simulink model "Phase 3 Onboard PFC Boost Charger-BMW i4 eDrive35 Gran Coupe Simulation"  (R2024b)
settings: Solver=VariableStepAuto  StartTime=0.0  StopTime=1  RelTol=1e-3
libraries: spsRMSLib x13, spsMeanLib x12, spsDiodeLib x9, spsCurrentMeasurementLib x5, spsMosfetLib x5, spsSeriesRLCBranchLib x5, spsVoltageMeasurementLib x5, slpidlib x2, spsPWMGeneratorDCDCLib x2, spsACVoltageSourceLib x1, spsLinearTransformerLib x1, sps_lib x1
settings Model: Creator=17249  LastModifiedBy=kunas
settings RTWCC: GPUComputeCapability=3.5

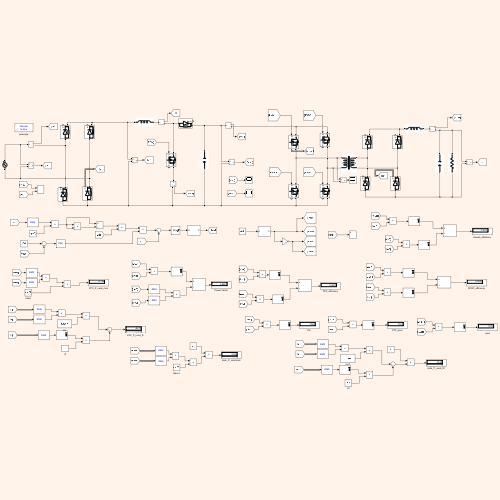
[thumbnail: Simulink's stored preview of the top-level diagram]
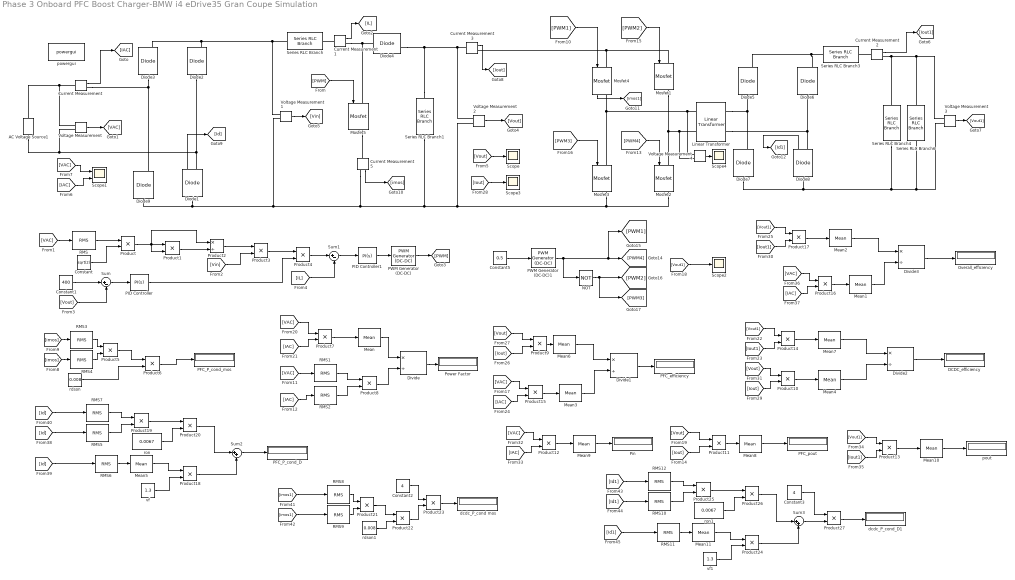
== system Phase 3 Onboard PFC Boost Charger-BMW i4 eDrive35 Gran Coupe Simulation ==
  AC Voltage Source1 : spsACVoltageSourceLib/AC Voltage Source  Amplitude=240  Phase=0  Frequency=60  SampleTime=0  Measurements=None  BusType=swing  Pref=10e3  Qref=0  Qmin=-inf  Qmax=+inf
  Constant : Constant  Value=sqrt(2)
  Constant1 : Constant  Value=400
  Constant2 : Constant  Value=4
  Constant3 : Constant  Value=4
  Constant5 : Constant  Value=0.5
  Current Measurement{,1..3,5} (5 alike) : spsCurrentMeasurementLib/Current Measurement  PhasorSimulation=off  OutputType=Complex  PSBequivalent=0
  DCDC_efficiency : Display
  Diode{1..4,9} (5 alike) : spsDiodeLib/Diode  Ron=0.0067  Lon=0  Vf=1.3  IC=0  UseSnubber=0  Rs=500  Cs=250e-9  Measurements=on
  Diode{5..8} (4 alike) : spsDiodeLib/Diode  Ron=0.0067  Lon=0  Vf=1.3  IC=0  UseSnubber=0  Rs=1e6  Cs=250e-9  Measurements=on
  Divide{,1..3} (4 alike) : Product  Inputs=*/  RndMeth=Zero  SaturateOnIntegerOverflow=on
  Linear Transformer : spsLinearTransformerLib/Linear Transformer  UNITS=SI  NominalPower=[ 8000 20000 ]  winding1=[400 1e-4 1e-6]  winding2=[400 1e-4 1e-6]  ThreeWindings=off  winding3=[3.15e+05 0.7938 0.084225]  RmLm=[1e6 1]  Measurements=None  DataType=on
  Mean{,1..11} (12 alike) : spsMeanLib/Mean  Freq=60  Vinit=0  Ts=0
  Mosfet{1..4} (4 alike) : spsMosfetLib/Mosfet  Ron=0.008  Lon=0  Rd=0.008  Vfd=3  IC=0  Rs=1e6  Cs=250e-9  Measurements=on
  Mosfet5 : spsMosfetLib/Mosfet  Ron=0.008  Lon=0  Rd=0.01  Vfd=3  IC=0  Rs=5000  Cs=250e-9  Measurements=on
  NOT : Logic  Operator=NOT  IconShape=distinctive  AllPortsSameDT=off  OutDataTypeStr=boolean
  Overall_efficiency : Display
  PFC_P_cond_D : Display
  PFC_P_cond_mos : Display
  PFC_efficiency : Display
  PFC_pout : Display
  PID Controller : slpidlib/PID Controller  Controller=PI  Form=Parallel  TimeDomain=Continuous-time  UseExternalTs=off  SampleTime=-1  IntegratorMethod=Forward Euler  FilterMethod=Forward Euler  ControllerParametersSource=internal  P=0.25  I=35  UseKiTs=off  D=0  UseExternalDerivativeSource=off  N=100  UseFilter=on  TunerSelectOption=Transfer Function Based (PID Tuner App)  InitialConditionSource=internal  InitialConditionForIntegrator=0  InitialConditionForFilter=0  DifferentiatorICPrevScaledInput=0  ExternalReset=none  TrackingMode=off  Kt=1  LimitOutput=off  SatLimitsSource=internal  UpperSaturationLimit=inf  LowerSaturationLimit=-inf  LinearizeAsGain=on  AntiWindupMode=none  Kb=1  LimitIntegrator=off  UpperIntegratorSaturationLimit=inf  LowerIntegratorSaturationLimit=-inf  POutMin=[]  POutMax=[]  IOutMin=[]  IOutMax=[]  DOutMin=[]  DOutMax=[]  NOutMin=[]  NOutMax=[]  SumOutMin=[]  SumOutMax=[]  SaturationOutMin=[]  SaturationOutMax=[]  PParamMin=[]  PParamMax=[]  IParamMin=[]  IParamMax=[]  DParamMin=[]  DParamMax=[]  NParamMin=[]  NParamMax=[]  KbParamMin=[]  KbParamMax=[]  KtParamMin=[]  KtParamMax=[]  KbOutMin=[]  KbOutMax=[]  KtOutMin=[]  KtOutMax=[]  IntegratorOutMin=[]  IntegratorOutMax=[]  FilterOutMin=[]  FilterOutMax=[]  SumI1OutMin=[]  SumI1OutMax=[]  SumI2OutMin=[]  SumI2OutMax=[]  SumI3OutMin=[]  SumI3OutMax=[]  SumI4OutMin=[]  SumI4OutMax=[]  SumDOutMin=[]  SumDOutMax=[]  DifferentiatorOutMin=[]  DifferentiatorOutMax=[]  FilterDiffOutCoefMin=[]  FilterDiffOutCoefMax=[]  ReciprocalOutMin=[]  ReciprocalOutMax=[]  SumDenOutMin=[]  SumDenOutMax=[]  SumNumOutMin=[]  SumNumOutMax=[]  DivideOutMin=[]  DivideOutMax=[]  UdiffTsProdOutMin=[]  UdiffTsProdOutMax=[]  NTsProdOutMin=[]  NTsProdOutMax=[]  UintegralTsProdOutMin=[]  UintegralTsProdOutMax=[]  UngainTsProdOutMin=[]  UngainTsProdOutMax=[]  ClampingZeroOutDataTypeStr=Inherit: Inherit via back propagation  ClampingZeroOutMin=[]  ClampingZeroOutMax=[]  FilterDenConstantOutDataTypeStr=Inherit: Inherit via back propagation  FilterDenConstantOutMin=[]  FilterDenConstantOutMax=[]  PCopyOutDataTypeStr=Inherit: Inherit via back propagation  PCopyOutMin=[]  PCopyOutMax=[]  NCopyOutDataTypeStr=Inherit: Inherit via back propagation  NCopyOutMin=[]  NCopyOutMax=[]  IntegratorContinuousStateAttributes=''  IntegratorStateMustResolveToSignalObject=off  IntegratorRTWStateStorageClass=Auto  FilterContinuousStateAttributes=''  FilterStateMustResolveToSignalObject=off  FilterRTWStateStorageClass=Auto  ParallelPVariant=InternalParameters  IdealPVariant=Disabled  IVariant=InternalParameters  DVariant=Disabled  IntegratorVariant=Continuous  SatVariant=Disabled  AWVariant=Passthrough  PCopyVariant=Disabled  TRVariant=Disabled  FdbkBlocksVariant=Forward  IdealPFdbkVariant=Disabled  SatFdbkVariant=Disabled  DerivativeFilterVariant=Disabled  NVariant=Disabled  NCopyVariant=Disabled_SignalSpec  FilterICVariant=Disabled  IntegratorICVariant=InternalICs  ExternalResetVariant=Disabled  TRSumVariant=Passthrough  SumFdbkVariant=Disabled  SumVariant=Sum_PI  TsampFilterVariant=InternalTs  TsampNgainVariant=Passthrough  TsampIntegralVariant=Disabled_SignalSpec  ExternalSaturationOutDataTypeStr=Inherit: Same as second input  DerivativeSourceVariant=Disabled  PreIntVariant=InternalPreInt
  PID Controller1 : slpidlib/PID Controller  Controller=PI  Form=Parallel  TimeDomain=Continuous-time  UseExternalTs=off  SampleTime=-1  IntegratorMethod=Forward Euler  FilterMethod=Forward Euler  ControllerParametersSource=internal  P=2000  I=0.25  UseKiTs=off  D=0  UseExternalDerivativeSource=off  N=100  UseFilter=on  TunerSelectOption=Transfer Function Based (PID Tuner App)  InitialConditionSource=internal  InitialConditionForIntegrator=0  InitialConditionForFilter=0  DifferentiatorICPrevScaledInput=0  ExternalReset=none  TrackingMode=off  Kt=1  LimitOutput=on  SatLimitsSource=internal  UpperSaturationLimit=0.95  LowerSaturationLimit=0  LinearizeAsGain=on  AntiWindupMode=none  Kb=1  LimitIntegrator=off  UpperIntegratorSaturationLimit=inf  LowerIntegratorSaturationLimit=-inf  POutMin=[]  POutMax=[]  IOutMin=[]  IOutMax=[]  DOutMin=[]  DOutMax=[]  NOutMin=[]  NOutMax=[]  SumOutMin=[]  SumOutMax=[]  SaturationOutMin=[]  SaturationOutMax=[]  PParamMin=[]  PParamMax=[]  IParamMin=[]  IParamMax=[]  DParamMin=[]  DParamMax=[]  NParamMin=[]  NParamMax=[]  KbParamMin=[]  KbParamMax=[]  KtParamMin=[]  KtParamMax=[]  KbOutMin=[]  KbOutMax=[]  KtOutMin=[]  KtOutMax=[]  IntegratorOutMin=[]  IntegratorOutMax=[]  FilterOutMin=[]  FilterOutMax=[]  SumI1OutMin=[]  SumI1OutMax=[]  SumI2OutMin=[]  SumI2OutMax=[]  SumI3OutMin=[]  SumI3OutMax=[]  SumI4OutMin=[]  SumI4OutMax=[]  SumDOutMin=[]  SumDOutMax=[]  DifferentiatorOutMin=[]  DifferentiatorOutMax=[]  FilterDiffOutCoefMin=[]  FilterDiffOutCoefMax=[]  ReciprocalOutMin=[]  ReciprocalOutMax=[]  SumDenOutMin=[]  SumDenOutMax=[]  SumNumOutMin=[]  SumNumOutMax=[]  DivideOutMin=[]  DivideOutMax=[]  UdiffTsProdOutMin=[]  UdiffTsProdOutMax=[]  NTsProdOutMin=[]  NTsProdOutMax=[]  UintegralTsProdOutMin=[]  UintegralTsProdOutMax=[]  UngainTsProdOutMin=[]  UngainTsProdOutMax=[]  ClampingZeroOutDataTypeStr=Inherit: Inherit via back propagation  ClampingZeroOutMin=[]  ClampingZeroOutMax=[]  FilterDenConstantOutDataTypeStr=Inherit: Inherit via back propagation  FilterDenConstantOutMin=[]  FilterDenConstantOutMax=[]  PCopyOutDataTypeStr=Inherit: Inherit via back propagation  PCopyOutMin=[]  PCopyOutMax=[]  NCopyOutDataTypeStr=Inherit: Inherit via back propagation  NCopyOutMin=[]  NCopyOutMax=[]  IntegratorContinuousStateAttributes=''  IntegratorStateMustResolveToSignalObject=off  IntegratorRTWStateStorageClass=Auto  FilterContinuousStateAttributes=''  FilterStateMustResolveToSignalObject=off  FilterRTWStateStorageClass=Auto  ParallelPVariant=InternalParameters  IdealPVariant=Disabled  IVariant=InternalParameters  DVariant=Disabled  IntegratorVariant=Continuous  SatVariant=Enabled  AWVariant=Passthrough  PCopyVariant=Disabled  TRVariant=Disabled  FdbkBlocksVariant=Forward  IdealPFdbkVariant=Disabled  SatFdbkVariant=Disabled  DerivativeFilterVariant=Disabled  NVariant=Disabled  NCopyVariant=Disabled_SignalSpec  FilterICVariant=Disabled  IntegratorICVariant=InternalICs  ExternalResetVariant=Disabled  TRSumVariant=Passthrough  SumFdbkVariant=Disabled  SumVariant=Sum_PI  TsampFilterVariant=InternalTs  TsampNgainVariant=Passthrough  TsampIntegralVariant=Disabled_SignalSpec  ExternalSaturationOutDataTypeStr=Inherit: Same as second input  DerivativeSourceVariant=Disabled  PreIntVariant=InternalPreInt
  PWM Generator (DC-DC) : spsPWMGeneratorDCDCLib/PWM Generator (DC-DC)  Fsw=65000  Ts=1e-6
  PWM Generator (DC-DC)1 : spsPWMGeneratorDCDCLib/PWM Generator (DC-DC)  Fsw=20000  Ts=0
  Pin : Display
  Power Factor : Display
  Product{,1,3..27} (27 alike) : Product
  Product2 : Product  Inputs=*/
  RMS{,3..12} (11 alike) : spsRMSLib/RMS  TrueRMS=on  Freq=60  RMSInit=240  Ts=0
  RMS1 : spsRMSLib/RMS  TrueRMS=on  Freq=60  RMSInit=120  Ts=0
  RMS2 : spsRMSLib/RMS  TrueRMS=on  Freq=60  RMSInit=120  Ts=0
  Scope{,2..4} (4 alike) : Scope
  Scope1 : Scope  NumInputPorts=2
  Series RLC Branch : spsSeriesRLCBranchLib/Series RLC Branch  LConnTagsString=__new0  RConnTagsString=__new0  BranchType=L  Resistance=1  Inductance=0.3e-3  SetiL0=off  InitialCurrent=0  Capacitance=1e-6  Setx0=off  InitialVoltage=0  Measurements=None
  Series RLC Branch1 : spsSeriesRLCBranchLib/Series RLC Branch  LConnTagsString=__new0  RConnTagsString=__new0  BranchType=C  Resistance=1  Inductance=0.3e-3  SetiL0=off  InitialCurrent=0  Capacitance=2000e-6  Setx0=off  InitialVoltage=0  Measurements=None
  Series RLC Branch3 : spsSeriesRLCBranchLib/Series RLC Branch  LConnTagsString=__new0  RConnTagsString=__new0  BranchType=L  Resistance=1  Inductance=2.5e-3  SetiL0=off  InitialCurrent=0  Capacitance=1e-6  Setx0=off  InitialVoltage=0  Measurements=None
  Series RLC Branch4 : spsSeriesRLCBranchLib/Series RLC Branch  LConnTagsString=__new0  RConnTagsString=__new0  BranchType=C  Resistance=1  Inductance=0.3e-3  SetiL0=off  InitialCurrent=0  Capacitance=100e-6  Setx0=off  InitialVoltage=0  Measurements=None
  Series RLC Branch6 : spsSeriesRLCBranchLib/Series RLC Branch  LConnTagsString=__new0  RConnTagsString=__new0  BranchType=R  Resistance=21.5  Inductance=0.3e-3  SetiL0=off  InitialCurrent=0  Capacitance=100e-6  Setx0=off  InitialVoltage=0  Measurements=None
  Sum : Sum  Inputs=|+-
  Sum1 : Sum  Inputs=|+-
  Sum2 : Sum  Inputs=|++
  Sum3 : Sum  Inputs=|++
  Voltage Measurement{,1..4} (5 alike) : spsVoltageMeasurementLib/Voltage Measurement  PhasorSimulation=off  OutputType=Complex  PSBequivalent=0
  dcdc_P_cond mos : Display
  dcdc_P_cond_D1 : Display
  pout : Display
  powergui : sps_lib/powergui  Priority=1  SimulationMode=Discrete  SampleTime=1e-6  frequency=60  Iterations=50  frequencyindice=0  Pbase=100e6  ErrMax=1e-4  UnitsV=kV  UnitsW=MW  buscounter=0  FunctionMessages=off  echomessages=off  EnableUseOfTLC=off  CurrentSourceSwitches=off  DisableSnubberDevices=off  DisableRonSwitches=off  DisableVfSwitches=off  DisplayEquations=off  AutomaticDiscreteSolvers=off  SolverType=Tustin/Backward Euler (TBE)  Interpol=off  ExternalGateDelay=off  methode=off  Ts=100  x0status=blocks  SPID=on  SwTol=0  HookPort=off  NonlinearTolerance=1e-4  nMaxIteration=100  ContinueOnMaxIteration=off  RestoreLinks=warning  ResistiveCurrentMeasurement=off  Frange=[0:2:500]  Ylog=off  Xlog=on  ShowGrid=off  save=off  variable=ZData  structure=0  ZoomFFT=off  StartTime=0.0  cycles=1  DisplayStyle=1  fundamental=60  FreqAxis=off  MaxFrequency=1000  frequencyindicesteady=1  RmsSteady=1  display=off
  rdson : Constant  Value=0.008
  rdson1 : Constant  Value=0.008
  ron : Constant  Value=0.0067
  ron1 : Constant  Value=0.0067
  vf : Constant  Value=1.3
  vf1 : Constant  Value=1.3
  wires:
  [VAC] -> Scope1/1
  [Iout] -> Scope3/1
  PWM Generator (DC-DC)1/1 -> [PWM1], [PWM4], NOT/1
  [PWM3] -> Mosfet3/1
  Voltage Measurement2/1 -> [Vout]
  Constant/1 -> Product/2
  [Vout] -> Sum/2
  [IL] -> Sum1/2
  [PWM4] -> Mosfet2/1
  Current Measurement1/1 -> [IL]
  Product4/1 -> Sum1/1
  [PWM2] -> Mosfet1/1
  [IAC] -> Scope1/2
  Constant5/1 -> PWM Generator (DC-DC)1/1
  Current Measurement3/1 -> [Iout]
  NOT/1 -> [PWM3], [PWM2]
  Product2/1 -> Product3/1
  Current Measurement2/1 -> [Iout1]
  Sum1/1 -> PID Controller1/1
  Voltage Measurement3/1 -> [Vout1]
  [VAC] -> RMS/1
  Voltage Measurement4/1 -> Scope4/1
  PID Controller1/1 -> PWM Generator (DC-DC)/1
  Voltage Measurement/1 -> [VAC]
  Product/1 -> Product2/1, Product1/2, Product1/1
  PWM Generator (DC-DC)/1 -> [PWM]
  RMS/1 -> Product/1
  [Vin] -> Product3/2
  Current Measurement/1 -> [IAC]
  [PWM] -> Mosfet5/1
  Sum/1 -> PID Controller/1
  PID Controller/1 -> Product4/2
  [PWM1] -> Mosfet4/1
  [Vout] -> Scope/1
  [Vout1] -> Scope2/1
  Constant1/1 -> Sum/1
  Voltage Measurement1/1 -> [Vin]
  Product1/1 -> Product2/2
  Product3/1 -> Product4/1
  rdson/1 -> Product6/2
  Product5/1 -> Product6/1
  Product6/1 -> PFC_P_cond_mos/1
  [Vout1] -> Product13/1
  Product13/1 -> Mean10/1
  Product10/1 -> Mean4/1
  Mean10/1 -> pout/1
  Mean8/1 -> PFC_pout/1
  [Vout] -> Product9/1
  [VAC] -> Product15/1
  [IAC] -> Product15/2
  Mean6/1 -> Divide1/1
  Mean3/1 -> Divide1/2
  Mean9/1 -> Pin/1
  [IAC] -> Product12/2
  Product9/1 -> Mean6/1
  [Iout1] -> Product13/2
  [VAC] -> Product12/1
  Product12/1 -> Mean9/1
  Divide1/1 -> PFC_efficiency/1
  Mean7/1 -> Divide2/1
  Product11/1 -> Mean8/1
  [Vout] -> Product11/1
  Product14/1 -> Mean7/1
  [Iout] -> Product9/2
  Divide2/1 -> DCDC_efficiency/1
  RMS2/1 -> Product8/2
  Product8/1 -> Divide/2
  [Vout1] -> Product14/1
  [Iout] -> Product11/2
  Product15/1 -> Mean3/1
  [IAC] -> Product7/2
  [Vout] -> Product10/1
  [Iout] -> Product10/2
  [VAC] -> Product7/1
  RMS1/1 -> Product8/1
  Product7/1 -> Mean/1
  [IAC] -> RMS2/1
  Divide/1 -> Power Factor/1
  [VAC] -> RMS1/1
  [Iout1] -> Product14/2
  Mean/1 -> Divide/1
  Mean4/1 -> Divide2/2
  [Iout1] -> Product17/2
  [Vout1] -> Product17/1
  Divide3/1 -> Overall_efficiency/1
  Product17/1 -> Mean2/1
  Mean2/1 -> Divide3/1
  Mean1/1 -> Divide3/2
  [VAC] -> Product16/1
  [IAC] -> Product16/2
  Product16/1 -> Mean1/1
  Current Measurement5/1 -> [imos]
  [imos] -> RMS3/1
  RMS3/1 -> Product5/1
  [imos] -> RMS4/1
  RMS4/1 -> Product5/2
  Diode1/1 -> [Id]
  [Id] -> RMS5/1
  [Id] -> RMS6/1
  RMS6/1 -> Mean5/1
  vf/1 -> Product18/2
  Mean5/1 -> Product18/1
  [Id] -> RMS7/1
  RMS7/1 -> Product19/1
  RMS5/1 -> Product19/2
  Product19/1 -> Product20/1
  ron/1 -> Product20/2
  Sum2/1 -> PFC_P_cond_D/1
  Product20/1 -> Sum2/1
  Product18/1 -> Sum2/2
  Mosfet4/1 -> [imos1]
  RMS9/1 -> Product21/2
  RMS8/1 -> Product21/1
  Product21/1 -> Product22/1
  [imos1] -> RMS8/1
  [imos1] -> RMS9/1
  rdson1/1 -> Product22/2
  Constant2/1 -> Product23/1
  Product22/1 -> Product23/2
  Product23/1 -> dcdc_P_cond mos/1
  vf1/1 -> Product24/2
  Product25/1 -> Product26/1
  RMS12/1 -> Product25/1
  Mean11/1 -> Product24/1
  ron1/1 -> Product26/2
  Product24/1 -> Sum3/2
  [Id1] -> RMS10/1
  Product26/1 -> Sum3/1
  RMS11/1 -> Mean11/1
  RMS10/1 -> Product25/2
  [Id1] -> RMS11/1
  Diode8/1 -> [Id1]
  [Id1] -> RMS12/1
  Sum3/1 -> Product27/2
  Product27/1 -> dcdc_P_cond_D1/1
  Constant3/1 -> Product27/1
  connections:
  Series RLC Branch1/LConn1 -- Diode4/RConn1 -- Current Measurement3/LConn1 -- Voltage Measurement2/LConn1
  Linear Transformer/RConn1 -- Diode5/LConn1 -- Diode7/RConn1
  Series RLC Branch4/RConn1 -- Voltage Measurement3/LConn2 -- Series RLC Branch6/RConn1 -- Diode8/LConn1 -- Diode7/LConn1
  Series RLC Branch3/LConn1 -- Diode6/RConn1 -- Diode5/RConn1
  Linear Transformer/LConn2 -- Mosfet2/LConn1 -- Mosfet1/RConn1 -- Voltage Measurement4/LConn2
  Current Measurement3/RConn1 -- Mosfet4/LConn1 -- Mosfet1/LConn1
  Current Measurement1/RConn1 -- Mosfet5/LConn1 -- Diode4/LConn1
  Current Measurement/LConn1 -- AC Voltage Source1/RConn1 -- Voltage Measurement/LConn1
  Current Measurement2/RConn1 -- Voltage Measurement3/LConn1 -- Series RLC Branch6/LConn1 -- Series RLC Branch4/LConn1
  Linear Transformer/LConn1 -- Mosfet4/RConn1 -- Mosfet3/LConn1 -- Voltage Measurement4/LConn1
  Current Measurement/RConn1 -- Diode9/RConn1 -- Diode3/LConn1
  Voltage Measurement1/LConn2 -- Mosfet3/RConn1 -- Mosfet2/RConn1 -- Voltage Measurement2/LConn2 -- Series RLC Branch1/RConn1 -- Current Measurement5/RConn1 -- Diode9/LConn1 -- Diode1/LConn1
  AC Voltage Source1/LConn1 -- Voltage Measurement/LConn2 -- Diode1/RConn1 -- Diode2/LConn1
  Linear Transformer/RConn2 -- Diode8/RConn1 -- Diode6/LConn1
  Current Measurement2/LConn1 -- Series RLC Branch3/RConn1
  Current Measurement1/LConn1 -- Series RLC Branch/RConn1
  Diode2/RConn1 -- Voltage Measurement1/LConn1 -- Series RLC Branch/LConn1 -- Diode3/RConn1
  Mosfet5/RConn1 -- Current Measurement5/LConn1
